simulink model "HeadwayLinearFede"  (R2020a)
settings: Solver=VariableStepAuto  StartTime=0.0  StopTime=3000  RelTol=1e-3
values from neighbouring files (symbols this model uses):
  A = eval(A)    [HeadwayFede.m]
  B = eval(B)    [HeadwayFede.m]
  K = lqr(A,B,Q,R)    [HeadwayFede.m]
  xe = [iq1_ref; id1_ref; iq2_ref; id2_ref; v_ref]    [HeadwayFede.m]
settings Model: Creator=Federico  LastModifiedBy=Federico

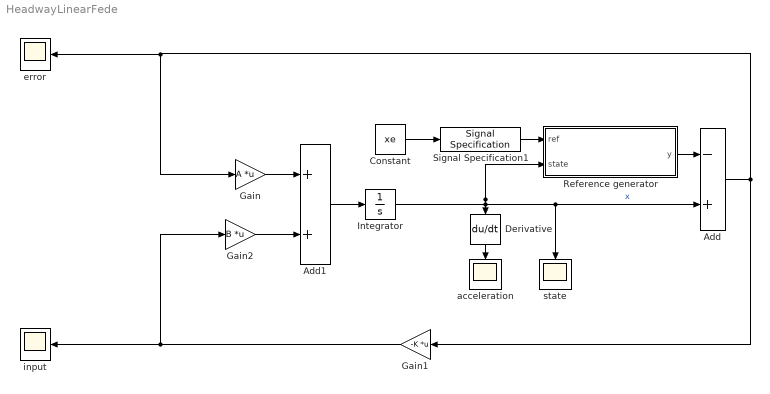
== system HeadwayLinearFede ==
  Add : Sum  Inputs=-+
  Add1 : Sum
  Constant : Constant  Value=xe
  Derivative : Derivative
  Gain : Gain  Gain=A  Multiplication=Matrix(K*u)
  Gain1 : Gain  Gain=-K  Multiplication=Matrix(K*u)
  Gain2 : Gain  Gain=B  Multiplication=Matrix(K*u)
  Integrator : Integrator  ContinuousStateAttributes='iq1.id1.iq2.id2.v'
  Reference generator : MATLAB Function  TreatAsAtomicUnit=on
  Signal Specification1 : SignalSpecification  Dimensions=5
  acceleration : Scope
  error : Scope
  input : Scope
  state : Scope
  wires:
  Gain/1 -> Add1/1
  Add1/1 -> Integrator/1
  Gain1/1 -> Gain2/1, input/1
  Gain2/1 -> Add1/2
  Add/1 -> Gain/1, error/1, Gain1/1
  Derivative/1 -> acceleration/1
  Constant/1 -> Signal Specification1/1
  Signal Specification1/1 -> Reference generator/1(ref)
  Integrator/1 -> Reference generator/2(state), Derivative/1, Add/2, state/1  "x"
  Reference generator/1(y) -> Add/1

== matlab function HeadwayLinearFede/Reference generator ==
  data: y output; ref input; state input
function y = fcn(ref, state)

y = zeros(5,1);

%current references
y(1) = ref(1);
y(2) = ref(2);
y(3) = ref(3);
y(4) = ref(4);

y(5) = state(5);


v_ref = ref(5); % velocity v_reference
tollerance = 0.1; %needed to obtain a good final beaviour
accFactor = 0.1; %with this you can change the slope of the velocity and so the acceleration

%Speed ramp profile
if y(5) < v_ref - tollerance
    y(5)=(y(5)+accFactor);
elseif y(5) > v_ref + tollerance
    y(5)=(y(5)-accFactor);
else
    y(5)=v_ref;
end
